simulink subsystem "Get_Traffic_by_Line"  (R2022b)
settings: Solver=VariableStepAuto  StartTime=0.0  StopTime=10.0  RelTol=1e-3
settings Model: Creator=user  LastModifiedBy=USER

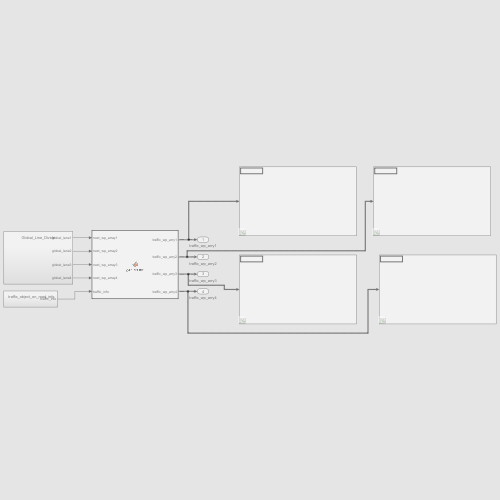
[thumbnail: Simulink's stored preview of the top-level diagram]
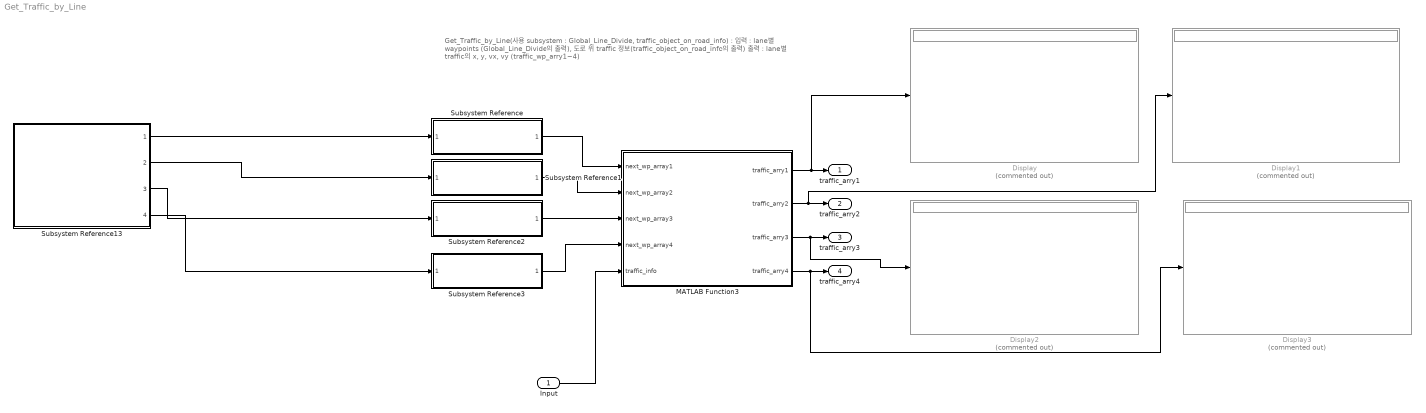
== system Get_Traffic_by_Line ==
  note: Get_Traffic_by_Line(사용 subsystem : Global_Line_Divide, traffic_object_on_road_info) :
      | 입력 : lane별 waypoints (Global_Line_Divide의 출력), 도로 위 traffic 정보(traffic_object_on_road_info의 출력)
      | 출력 : lane별 traffic의 x, y, vx, vy (traffic_wp_arry1~4)
  Input : Inport
  Display{,1..3} (4 alike) : Display  Commented=on
  MATLAB Function3 : MATLAB Function  TreatAsAtomicUnit=on
  Subsystem Reference{,1..3} (4 alike) : Subsystem  ReferencedSubsystem=global_to_local_waypoint_junho
  Subsystem Reference13 : Subsystem  ReferencedSubsystem=Global_Line_Divide
  traffic_arry1 : Outport
  traffic_arry2 : Outport  Port=2
  traffic_arry3 : Outport  Port=3
  traffic_arry4 : Outport  Port=4
  wires:
  MATLAB Function3/3(traffic_arry3) -> Display2/1, traffic_arry3/1
  MATLAB Function3/2(traffic_arry2) -> Display1/1, traffic_arry2/1
  MATLAB Function3/4(traffic_arry4) -> Display3/1, traffic_arry4/1
  MATLAB Function3/1(traffic_arry1) -> Display/1, traffic_arry1/1
  Subsystem Reference/1 -> MATLAB Function3/1(next_wp_array1)
  Subsystem Reference13/1 -> Subsystem Reference/1
  Subsystem Reference13/2 -> Subsystem Reference1/1
  Subsystem Reference1/1 -> MATLAB Function3/2(next_wp_array2)
  Subsystem Reference2/1 -> MATLAB Function3/3(next_wp_array3)
  Subsystem Reference13/3 -> Subsystem Reference2/1
  Subsystem Reference3/1 -> MATLAB Function3/4(next_wp_array4)
  Subsystem Reference13/4 -> Subsystem Reference3/1
  Input/1 -> MATLAB Function3/5(traffic_info)

== matlab function Get_Traffic_by_Line/MATLAB Function3 ==
  settings: sampleTime=0.001
  data: next_wp_array1 input; next_wp_array2 input; next_wp_array3 input; next_wp_array4 input; traffic_arry1 output size=[8 4]; traffic_info input; traffic_arry2 output size=[8 4]; traffic_arry3 output size=[8 4]; traffic_arry4 output size=[8 4]
function [traffic_arry1, traffic_arry2, traffic_arry3, traffic_arry4] = get_traffic(next_wp_array1, next_wp_array2, next_wp_array3, next_wp_array4, traffic_info)
    tolerance = 3; % 트래픽 위치에 대한 오차 허용 범위

    % Initialize traffic waypoints array with NaNs (size 10x4 to limit maximum size)
    coder.varsize('traffic_arry1', [8, 4]);  % 행은 8로 설정, 열은 4로 고정
    traffic_arry1 = zeros(0,4);
    coder.varsize('traffic_arry2', [8, 4]);  % 행은 8로 설정, 열은 4로 고정
    traffic_arry2 = zeros(0,4);
    coder.varsize('traffic_arry3', [8, 4]);  % 행은 8로 설정, 열은 4로 고정
    traffic_arry3 = zeros(0,4);
    coder.varsize('traffic_arry4', [8, 4]);  % 행은 8로 설정, 열은 4로 고정
    traffic_arry4 = zeros(0,4);

    % 트래픽 정보를 각 lane의 waypoints와 비교하여 저장
    for i = 1:size(traffic_info, 1) % 각 트래픽 정보에 대해 반복
        traffic_x = traffic_info(i, 1);
        traffic_y = traffic_info(i, 2);
        traffic_v = traffic_info(i, 3);
        traffic_dis = traffic_info(i, 4);

        % 각 lane의 waypoints와 트래픽 위치 비교 (오차 tolerance 범위 내)
        if is_within_tolerance(traffic_x, traffic_y, next_wp_array1, tolerance)
            traffic_arry1 = add_to_traffic_array(traffic_arry1, [traffic_x, traffic_y, traffic_v, traffic_dis]);
        elseif is_within_tolerance(traffic_x, traffic_y, next_wp_array2, tolerance)
            traffic_arry2 = add_to_traffic_array(traffic_arry2, [traffic_x, traffic_y, traffic_v, traffic_dis]);
        elseif is_within_tolerance(traffic_x, traffic_y, next_wp_array3, tolerance)
            traffic_arry3 = add_to_traffic_array(traffic_arry3, [traffic_x, traffic_y, traffic_v, traffic_dis]);
        elseif is_within_tolerance(traffic_x, traffic_y, next_wp_array4, tolerance)
            traffic_arry4 = add_to_traffic_array(traffic_arry4, [traffic_x, traffic_y, traffic_v, traffic_dis]);
        end
    end
end

% 트래픽 좌표가 해당 lane의 waypoints와 오차 tolerance 범위 내에 있는지 확인하는 함수
function is_within = is_within_tolerance(traffic_x, traffic_y, waypoints, tolerance)
    distances = sqrt((waypoints(:, 1) - traffic_x).^2 + (waypoints(:, 2) - traffic_y).^2);
    is_within = any(distances <= tolerance); % 오차 tolerance 이내에 있는지 확인
end

% 트래픽 정보를 해당 lane array에 추가하는 함수
function updated_array = add_to_traffic_array(traffic_array, traffic_data)
    % 배열의 크기를 제한 (최대 8x4)
    if size(traffic_array, 1) < 8
        % 현재 배열에 행 추가
        traffic_array = [traffic_array; traffic_data];
    end
    updated_array = traffic_array;
end
